simulink model "SimulinkP8_2"  (R2018b)
settings: Solver=VariableStepAuto  StartTime=0.0  StopTime=30  RelTol=1e-3
values from neighbouring files (symbols this model uses):
  A = [ 0 1; 0 -3 ]    [Problema8_2.m]
  B = [ 0; 2]    [Problema8_2.m]
  C1 = [ 1 0 ]    [Problema8_2.m]
  C2 = [ 0 1 ]    [Problema8_2.m]
  Ca = [ 1 0; 0 1 ]    [Problema8_2.m]
  Da = [ 0; 0 ]    [Problema8_2.m]
  h = 0.1    [Problema8_2.m]
  L = [0 1] * inv(Wc) * (phi^2 + p1 * phi + p2 * eye(2))    [Problema8_2.m]
  Lc = Ganho_DC/( C * inv(eye(2) - phi_cl ) * gama )    [Problema8_2.m]
  p_load = 0.5    [Problema8_2.m]
  t_pert = 20    [Problema8_2.m]
  t_ref = 10    [Problema8_2.m]
  x0 = [ 1; 1]    [Problema8_2.m]
settings Model: Creator=root  LastModifiedBy=root

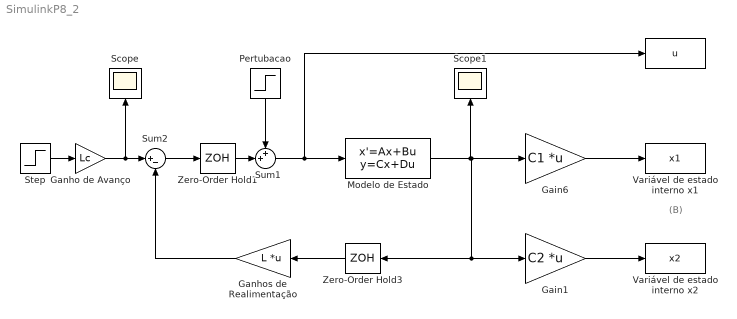
== system SimulinkP8_2 ==
  note: (B)
  " " : ToWorkspace  VariableName=u  SaveFormat=Structure With Time  SampleTime=-1
  Gain1 : Gain  Gain=C2  Multiplication=Matrix(K*u)
  Gain6 : Gain  Gain=C1  Multiplication=Matrix(K*u)
  Ganho de Avanço : Gain  Gain=Lc
  Ganhos de Realimentação : Gain  Gain=L  Multiplication=Matrix(K*u)
  Modelo de Estado : StateSpace  A=A  B=B  C=Ca  D=Da  InitialCondition=x0
  Pertubacao : Step  Time=t_pert  After=p_load  SampleTime=0
  Scope : Scope
  Scope1 : Scope
  Step : Step  Time=t_ref  SampleTime=0
  Sum1 : Sum  Inputs=++|
  Sum2 : Sum  Inputs=|+-
  Variável de estado interno x1 : ToWorkspace  VariableName=x1  SaveFormat=Structure With Time  SampleTime=-1
  Variável de estado interno x2 : ToWorkspace  VariableName=x2  SaveFormat=Structure With Time  SampleTime=-1
  Zero-Order Hold1 : ZeroOrderHold  SampleTime=h
  Zero-Order Hold3 : ZeroOrderHold  SampleTime=h
  wires:
  Gain1/1 -> Variável de estado interno x2/1
  Ganho de Avanço/1 -> Sum2/1, Scope/1
  Zero-Order Hold3/1 -> Ganhos de Realimentação/1
  Ganhos de Realimentação/1 -> Sum2/2
  Gain6/1 -> Variável de estado interno x1/1
  Step/1 -> Ganho de Avanço/1
  Sum2/1 -> Zero-Order Hold1/1
  Modelo de Estado/1 -> Gain6/1, Gain1/1, Zero-Order Hold3/1, Scope1/1
  Zero-Order Hold1/1 -> Sum1/2
  Sum1/1 -> " "/1, Modelo de Estado/1
  Pertubacao/1 -> Sum1/1
